simulink model "con_lac_don"  (R2023a)
settings: Solver=ode4  StartTime=0.0  StopTime=10.0  FixedStep=0.001  RelTol=1e-3
settings Model: Creator=VINH  LastModifiedBy=VINH

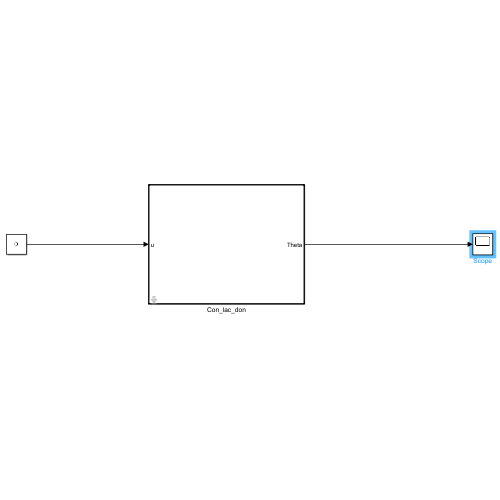
[thumbnail: Simulink's stored preview of the top-level diagram]
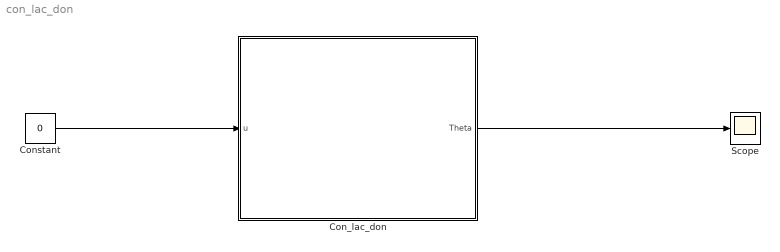
== system con_lac_don ==
  Con_lac_don : Subsystem  TreatAsAtomicUnit=on  mask{g=9.81, l=0.2, m=0.5, B=0, theta_init=0.5, theta_dot_init=0}
      mask prompts: g "Gia toc trong truong (m/s2)"; l "Chieu dai con lac (m)"; m "Khoi luong vat nang (kg)"; B "He so ma sat"; theta_init "Goc ban dau (rad)"; theta_dot_init "Van toc goc ban dau (rad/s)"
  Constant : Constant  Value=0
  Scope : Scope
  wires:
  Constant/1 -> Con_lac_don/1(u)
  Con_lac_don/1(Theta) -> Scope/1

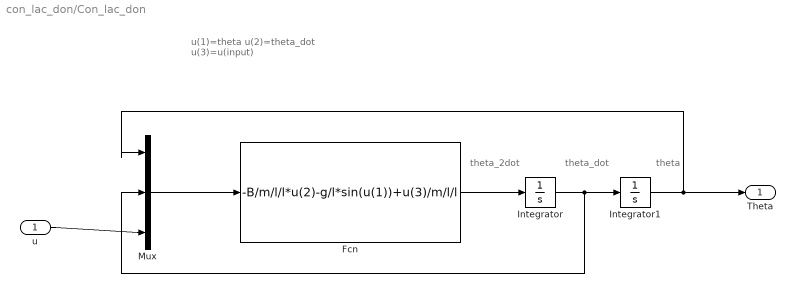
== system con_lac_don/Con_lac_don ==
  note: theta
  note: theta_dot
  note: theta_2dot
  note: u(1)=theta
      | u(2)=theta_dot
      | u(3)=u(input)
  u : Inport
  Fcn : Fcn  Expr=-B/m/l/l*u(2)-g/l*sin(u(1))+u(3)/m/l/l
  Integrator : Integrator  InitialCondition=theta_dot_init
  Integrator1 : Integrator  InitialCondition=theta_init
  Mux : Mux  Inputs=3
  Theta : Outport
  wires:
  u/1 -> Mux/3
  Integrator1/1 -> Theta/1, Mux/1
  Integrator/1 -> Mux/2, Integrator1/1
  Mux/1 -> Fcn/1
  Fcn/1 -> Integrator/1
